simulink model "Demo"  (R2021a)
settings: Solver=FixedStepDiscrete  StartTime=0.0  StopTime=10  FixedStep=0.005  RelTol=1e-3  EnableMultiTasking=on
PreLoadFcn:
  | disp(pwd)
PostLoadFcn:
  | c2000demoscallback(1)
undefined symbols (not defined in the file or in its folder): CommandConstEnable, CommandData, FrameData, MailBoxRx, MailBoxTx, SCIAReceivedComplete, StatusConstClose, StatusConstClosed, StatusConstError, StatusConstHoming, StatusConstIdle, StatusConstPaused, StatusConstReady, StatusConstReset, StatusConstRunning, StatusConstStart, StatusConstStopped, StatusData
libraries: simulink x28, c280xlib x19, idelinklib_common x16, c2000lib x1, pid_lib x1, c2833xlib x1
(part 1 of 3)
settings Model: DataDictionary=DataD1.sldd  EnableAccessToBaseWorkspace=off  ExtModeTrigDuration=8  OrderedModelArguments=off  Creator=The MathWorks Inc.  LastModifiedBy=1
settings SolverCC: AlgebraicLoopSolver=TrustRegion
settings DataIOCC: LimitDataPoints=on  SaveFormat=Array  SignalLoggingSaveFormat=ModelDataLogs  SaveOutput=off  SaveTime=off  ReturnWorkspaceOutputs=off  SignalLoggingName=sigsOut
settings OptimizationCC: DefaultParameterBehavior=Inlined  DefaultUnderspecifiedDataType=single  PassReuseOutputArgsAs=Individual arguments  ExpressionDepthLimit=2147483647  InitFltsAndDblsToZero=on  LifeSpan=inf  MaxStackSize=512  EfficientTunableParamExpr=on
settings DebuggingCC: UnderspecifiedInitializationDetection=Classic  MergeDetectMultiDrivingBlocksExec=none  CheckExecutionContextPreStartOutputMsg=on  SignalResolutionControl=TryResolveAllWithWarning  MultiTaskDSMMsg=warning  MultiTaskCondExecSysMsg=none  SigSpecEnsureSampleTimeMsg=none  FcnCallInpInsideContextMsg=warning  StateNameClashWarn=warning  SFUnexpectedBacktrackingDiag=warning  SFNoUnconditionalDefaultTransitionDiag=warning  SFExecutionAtInitializationDiag=none  SFMachineParentedDataDiag=warning  ArithmeticOperatorsInVariantConditions=warning
settings HardwareCC: ProdBitPerChar=16  ProdBitPerInt=16  ProdBitPerPointer=32  ProdBitPerSizeT=32  ProdBitPerPtrDiffT=32  ProdLargestAtomicInteger=Integer  ProdLargestAtomicFloat=None  ProdWordSize=16  ProdLongLongMode=on  ProdHWDeviceType=Texas Instruments->C2000  TargetBitPerChar=16  TargetBitPerInt=16  TargetLargestAtomicInteger=Integer  TargetIntDivRoundTo=Zero  TargetEndianess=LittleEndian  TargetWordSize=16  TargetHWDeviceType=Texas Instruments->C2000  ProdEqTarget=off
settings ModelReferenceCC: UpdateModelReferenceTargets=IfOutOfDate  PropagateSignalLabelsOutOfModel=off
settings SFSimCC: SimUseLocalCustomCode=off  MATLABDynamicMemAlloc=off  CustomCodeUndefinedFunction=UseInterfaceOnly
settings RTWCC: SystemTargetFile=ert.tlc  HardwareBoard=TI Delfino F2833x  TemplateMakefile=ert_default_tmf  GenerateReport=on  RTWUseLocalCustomCode=off  Toolchain=Texas Instruments Code Composer Studio (C2000)  IncludeHyperlinkInReport=on  LaunchReport=on  GenerateTraceInfo=on  GenerateTraceReportSl=on  GenerateTraceReportSf=on  GenerateWebview=on
settings CodeAppCC: IgnoreCustomStorageClasses=off  SimulinkDataObjDesc=on  SFDataObjDesc=on  CustomSymbolStrType=$N$R$M  InsertBlockDesc=on  StateflowObjectComments=on  MATLABSourceComments=on  InternalIdentifier=Classic
settings ERTTargetCC: CodeReplacementLibrary=TI C28x  MultiwordLength=2048  ParMdlRefBuildCompliant=off  CPPClassGenCompliant=off  ConvertIfToSwitch=off  SuppressUnreachableDefaultCases=off
settings ConfigComp: CovMetricSettings=dw  CovSaveCumulativeToWorkspaceVar=on  CovSaveSingleToWorkspaceVar=on  CovExternalEMLEnable=off  CovSFcnEnable=off  PSAutoStubLUT=on

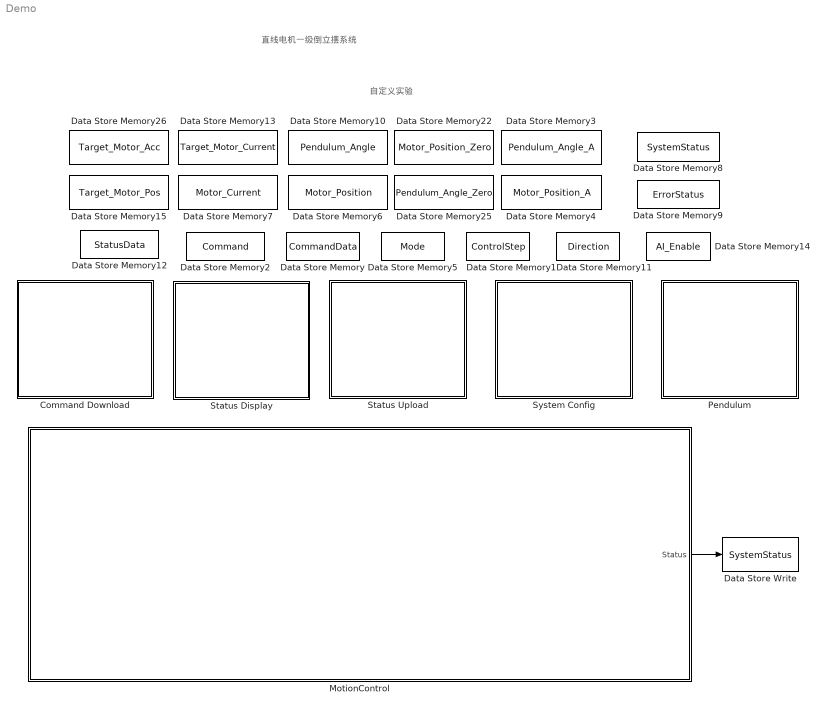
== system Demo ==
  note: 直线电机一级倒立摆系统
  note: 自定义实验
  Command Download : Subsystem  TreatAsAtomicUnit=on
  Data Store Memory11 : DataStoreMemory  DataStoreName=Direction  ReadBeforeWriteMsg=warning  WriteAfterWriteMsg=warning  WriteAfterReadMsg=warning  ShowAdditionalParam=off
  Data Store Memory14 : DataStoreMemory  DataStoreName=AI_Enable  ReadBeforeWriteMsg=warning  WriteAfterWriteMsg=warning  WriteAfterReadMsg=warning  InitialValue=1  ShowAdditionalParam=off  OutDataTypeStr=uint16
  Data Store Memory8 : DataStoreMemory  DataStoreName=SystemStatus  ReadBeforeWriteMsg=warning  WriteAfterWriteMsg=warning  WriteAfterReadMsg=warning  ShowAdditionalParam=off  OutDataTypeStr=uint16
  Data Store Memory9 : DataStoreMemory  DataStoreName=ErrorStatus  ReadBeforeWriteMsg=warning  WriteAfterWriteMsg=warning  WriteAfterReadMsg=warning  ShowAdditionalParam=off  OutDataTypeStr=uint16
  Data Store Write : DataStoreWrite  DataStoreName=SystemStatus  IndexOptions=Index vector (dialog)  Indices=1  OutputSizes=1
  Data Store Memory : DataStoreMemory  DataStoreName=CommandData  ReadBeforeWriteMsg=warning  WriteAfterWriteMsg=warning  WriteAfterReadMsg=warning  InitialValue=zeros(1,8)  ShowAdditionalParam=off  OutDataTypeStr=double
  Data Store Memory1 : DataStoreMemory  DataStoreName=ControlStep  ReadBeforeWriteMsg=warning  WriteAfterWriteMsg=warning  WriteAfterReadMsg=warning  ShowAdditionalParam=off  OutDataTypeStr=uint16
  Data Store Memory10 : DataStoreMemory  DataStoreName=Pendulum_Angle  ReadBeforeWriteMsg=warning  WriteAfterWriteMsg=warning  WriteAfterReadMsg=warning  ShowAdditionalParam=off  OutDataTypeStr=double
  Data Store Memory12 : DataStoreMemory  DataStoreName=StatusData  ReadBeforeWriteMsg=warning  WriteAfterWriteMsg=warning  WriteAfterReadMsg=warning  InitialValue=[0 0 0 0 0 0 0 0]  ShowAdditionalParam=off
  Data Store Memory13 : DataStoreMemory  DataStoreName=Target_Motor_Current  ReadBeforeWriteMsg=warning  WriteAfterWriteMsg=warning  WriteAfterReadMsg=warning  ShowAdditionalParam=off
  Data Store Memory15 : DataStoreMemory  DataStoreName=Target_Motor_Pos  ReadBeforeWriteMsg=warning  WriteAfterWriteMsg=warning  WriteAfterReadMsg=warning  ShowAdditionalParam=off
  Data Store Memory2 : DataStoreMemory  DataStoreName=Command  ReadBeforeWriteMsg=warning  WriteAfterWriteMsg=warning  WriteAfterReadMsg=warning  ShowAdditionalParam=off  OutDataTypeStr=uint16
  Data Store Memory22 : DataStoreMemory  DataStoreName=Motor_Position_Zero  ReadBeforeWriteMsg=warning  WriteAfterWriteMsg=warning  WriteAfterReadMsg=warning  ShowAdditionalParam=off  OutDataTypeStr=double
  Data Store Memory25 : DataStoreMemory  DataStoreName=Pendulum_Angle_Zero  ReadBeforeWriteMsg=warning  WriteAfterWriteMsg=warning  WriteAfterReadMsg=warning  ShowAdditionalParam=off  OutDataTypeStr=double
  Data Store Memory26 : DataStoreMemory  DataStoreName=Target_Motor_Acc  ReadBeforeWriteMsg=warning  WriteAfterWriteMsg=warning  WriteAfterReadMsg=warning  ShowAdditionalParam=off
  Data Store Memory3 : DataStoreMemory  DataStoreName=Pendulum_Angle_A  ReadBeforeWriteMsg=warning  WriteAfterWriteMsg=warning  WriteAfterReadMsg=warning  ShowAdditionalParam=off  OutDataTypeStr=double
  Data Store Memory4 : DataStoreMemory  DataStoreName=Motor_Position_A  ReadBeforeWriteMsg=warning  WriteAfterWriteMsg=warning  WriteAfterReadMsg=warning  ShowAdditionalParam=off  OutDataTypeStr=double
  Data Store Memory5 : DataStoreMemory  DataStoreName=Mode  ReadBeforeWriteMsg=warning  WriteAfterWriteMsg=warning  WriteAfterReadMsg=warning  ShowAdditionalParam=off  OutDataTypeStr=uint16
  Data Store Memory6 : DataStoreMemory  DataStoreName=Motor_Position  ReadBeforeWriteMsg=warning  WriteAfterWriteMsg=warning  WriteAfterReadMsg=warning  ShowAdditionalParam=off  OutDataTypeStr=double
  Data Store Memory7 : DataStoreMemory  DataStoreName=Motor_Current  ReadBeforeWriteMsg=warning  WriteAfterWriteMsg=warning  WriteAfterReadMsg=warning  ShowAdditionalParam=off
  MotionControl : Stateflow chart  TreatAsAtomicUnit=on
  Pendulum : Subsystem
  Status Display : Subsystem  TreatAsAtomicUnit=on
      settings: RTWSystemCode=Nonreusable function
  Status Upload : Subsystem  TreatAsAtomicUnit=on
  System Config : Subsystem  TreatAsAtomicUnit=on
  wires:
  MotionControl/1(Status) -> Data Store Write/1

== system Demo/Command Download ==
  Data Store Memory12 : DataStoreMemory  DataStoreName=FrameData  ReadBeforeWriteMsg=warning  WriteAfterWriteMsg=warning  WriteAfterReadMsg=warning  InitialValue=zeros(1,17)  ShowAdditionalParam=off  OutDataTypeStr=uint16
  SCIA_Interrupt : c2000lib/Scheduling/C28x Hardware Interrupt  irqnumbers=9  pienumbers=1  irqpriorities=0  irqpreempts=0  showinput=off  dspchiptype=C280X
      settings: SourceProductBaseCode=TIC2000
  SCIA_RX_Process : Subsystem  TreatAsAtomicUnit=on
  wires:
  SCIA_Interrupt/1 -> SCIA_RX_Process/Trigger

== system Demo/MotionControl/Close ==
  f : TriggerPort  TriggerType=function-call  VariantControl=(inherit)
      settings: CopyFcn=Stateflow.SLINSF.SimulinkMan.removeBlockPreDeleteFcn  PreDeleteFcn=Stateflow.SLINSF.SimulinkMan.unsafePredeleteFcn
  Constant : Constant  OutDataTypeStr=uint16
  Constant1 : Constant  Value=0
  Constant2 : Constant  Value=0  OutDataTypeStr=uint16
  Constant5 : Constant  Value=StatusConstIdle
  Data Store Write : DataStoreWrite  DataStoreName=AI_Enable  IndexOptions=Index vector (dialog)  Indices=1  OutputSizes=1
  Data Store Write1 : DataStoreWrite  DataStoreName=Target_Motor_Current  IndexOptions=Index vector (dialog)  Indices=1  OutputSizes=1
  Data Store Write2 : DataStoreWrite  DataStoreName=Target_Motor_Acc  IndexOptions=Index vector (dialog)  Indices=1  OutputSizes=1
  Data Store Write3 : DataStoreWrite  DataStoreName=Mode  IndexOptions=Index vector (dialog)  Indices=1  OutputSizes=1
  MO : Constant  Value=[hex2dec('4F4D') 0 0 0]  OutDataTypeStr=uint16
  eCANA Transmit : Subsystem  TreatAsAtomicUnit=on  mask(eCANA Transimit Blocks){MailBoxTx=1, MailBoxRx=4}
      mask help: eCANA MailBox Transimit
      mask DialogControl ParameterGroup Prompt: Parameter Setting
  Status : Outport  OutDataTypeStr=uint16  PortDimensions=[1 1]  VectorParamsAs1DForOutWhenUnconnected=off
  wires:
  Constant1/1 -> Data Store Write2/1, Data Store Write1/1
  Constant5/1 -> Status/1
  Constant/1 -> Data Store Write/1
  MO/1 -> eCANA Transmit/1(DataTx)
  Constant2/1 -> Data Store Write3/1

== system Demo/MotionControl/Home ==
  f : TriggerPort  TriggerType=function-call  VariantControl=(inherit)
      settings: CopyFcn=Stateflow.SLINSF.SimulinkMan.removeBlockPreDeleteFcn  PreDeleteFcn=Stateflow.SLINSF.SimulinkMan.unsafePredeleteFcn
  Add : Sum
  Compare To Constant1 : simulink/Logic and Bit Operations/Compare To Constant  relop=>=  const=uint16(15)  OutDataTypeStr=boolean
  Constant : Constant  Value=StatusConstHoming
  Constant1 : Constant  Value=StatusConstReady
  Data Store Read2 : DataStoreRead  DataStoreName=ControlStep  IndexOptions=Index vector (dialog)  Indices=1  OutputSizes=1
  PX : Subsystem  TreatAsAtomicUnit=on
  ResetAngle : Subsystem  TreatAsAtomicUnit=on
  Switch : Switch  Criteria=u2 > Threshold  Threshold=uint16(0)
  Switch Case : SwitchCase  CaseConditions={1,2,3,4}
  TForAI0 : Subsystem  TreatAsAtomicUnit=on
  TForAI1 : Subsystem  TreatAsAtomicUnit=on
  Status : Outport  OutDataTypeStr=uint16  PortDimensions=1
  wires:
  Switch Case/2 -> TForAI1/Action
  Constant/1 -> Add/1
  Switch Case/1 -> ResetAngle/Action
  Compare To Constant1/1 -> Switch/2
  Data Store Read2/1 -> Switch Case/1, Add/2, Compare To Constant1/1
  Add/1 -> Switch/3
  Constant1/1 -> Switch/1
  Switch Case/3 -> PX/Action
  Switch/1 -> Status/1
  Switch Case/4 -> TForAI0/Action

== system Demo/MotionControl/Idle ==
  f : TriggerPort  TriggerType=function-call  VariantControl=(inherit)
      settings: CopyFcn=Stateflow.SLINSF.SimulinkMan.removeBlockPreDeleteFcn  PreDeleteFcn=Stateflow.SLINSF.SimulinkMan.unsafePredeleteFcn
  Constant4 : Constant  Value=StatusConstReset
  Constant5 : Constant  Value=StatusConstStart
  Constant6 : Constant  Value=StatusConstIdle
  Data Store Read : DataStoreRead  DataStoreName=Command  IndexOptions=Index vector (dialog)  Indices=1  OutputSizes=1
  Index Vector : MultiPortSwitch  DataPortOrder=Specify indices  Inputs=1  DataPortIndices={CommandConstStart,CommandConstReset}  DataPortForDefault=Additional data port  DiagnosticForDefault=None
  Status : Outport  OutDataTypeStr=uint16  PortDimensions=[1 1]
  wires:
  Index Vector/1 -> Status/1
  Constant4/1 -> Index Vector/3
  Constant5/1 -> Index Vector/2
  Data Store Read/1 -> Index Vector/1
  Constant6/1 -> Index Vector/4

== system Demo/MotionControl/Initial ==
  f : TriggerPort  TriggerType=function-call  VariantControl=(inherit)
      settings: CopyFcn=Stateflow.SLINSF.SimulinkMan.removeBlockPreDeleteFcn  PreDeleteFcn=Stateflow.SLINSF.SimulinkMan.unsafePredeleteFcn
  Bus Assignment : BusAssignment  Priority=1  AssignedSignals=MailBoxTx,MailBoxRx
  Bus Assignment1 : BusAssignment  Priority=1  Commented=on  AssignedSignals=MailBoxTx,MailBoxRx
  Constant1 : Constant  Value=4  OutDataTypeStr=uint16  SampleTime=-1
  Constant2 : Constant  OutDataTypeStr=uint16  SampleTime=-1
  Constant3 : Constant  Commented=on  Value=5  OutDataTypeStr=uint16  SampleTime=-1
  Constant4 : Constant  Commented=on  Value=2  OutDataTypeStr=uint16  SampleTime=-1
  Data Store Read : DataStoreRead  DataStoreName=CanMsgA  IndexOptions=Index vector (dialog)  Indices=1  OutputSizes=1
  Data Store Read1 : DataStoreRead  Commented=on  DataStoreName=CanMsgA1  IndexOptions=Index vector (dialog)  Indices=1  OutputSizes=1
  Data Store Write : DataStoreWrite  DataStoreName=CanMsgA  IndexOptions=Index vector (dialog)  Indices=1  OutputSizes=1
  Data Store Write1 : DataStoreWrite  Commented=on  DataStoreName=CanMsgA1  IndexOptions=Index vector (dialog)  Indices=1  OutputSizes=1
  wires:
  Constant2/1 -> Bus Assignment/2
  Constant1/1 -> Bus Assignment/3
  Bus Assignment/1 -> Data Store Write/1
  Data Store Read/1 -> Bus Assignment/1
  Data Store Read1/1 -> Bus Assignment1/1
  Bus Assignment1/1 -> Data Store Write1/1
  Constant3/1 -> Bus Assignment1/3
  Constant4/1 -> Bus Assignment1/2

== system Demo/MotionControl/Ready ==
  f : TriggerPort  TriggerType=function-call  VariantControl=(inherit)
      settings: CopyFcn=Stateflow.SLINSF.SimulinkMan.removeBlockPreDeleteFcn  PreDeleteFcn=Stateflow.SLINSF.SimulinkMan.unsafePredeleteFcn
  Constant1 : Constant  Value=StatusConstHoming
  Constant2 : Constant  Value=StatusConstRunning
  Constant3 : Constant  Value=StatusConstReady
  Constant4 : Constant  Value=StatusConstClose
  Data Store Read : DataStoreRead  DataStoreName=Command  IndexOptions=Index vector (dialog)  Indices=1  OutputSizes=1
  Multiport Switch : MultiPortSwitch  DataPortOrder=Specify indices  DataPortIndices={CommandConstHome,CommandConstRun,CommandConstDisable}  DataPortForDefault=Additional data port  DiagnosticForDefault=None
  Status : Outport  OutDataTypeStr=uint16  PortDimensions=1
  wires:
  Data Store Read/1 -> Multiport Switch/1
  Constant2/1 -> Multiport Switch/3
  Constant1/1 -> Multiport Switch/2
  Multiport Switch/1 -> Status/1
  Constant3/1 -> Multiport Switch/5
  Constant4/1 -> Multiport Switch/4

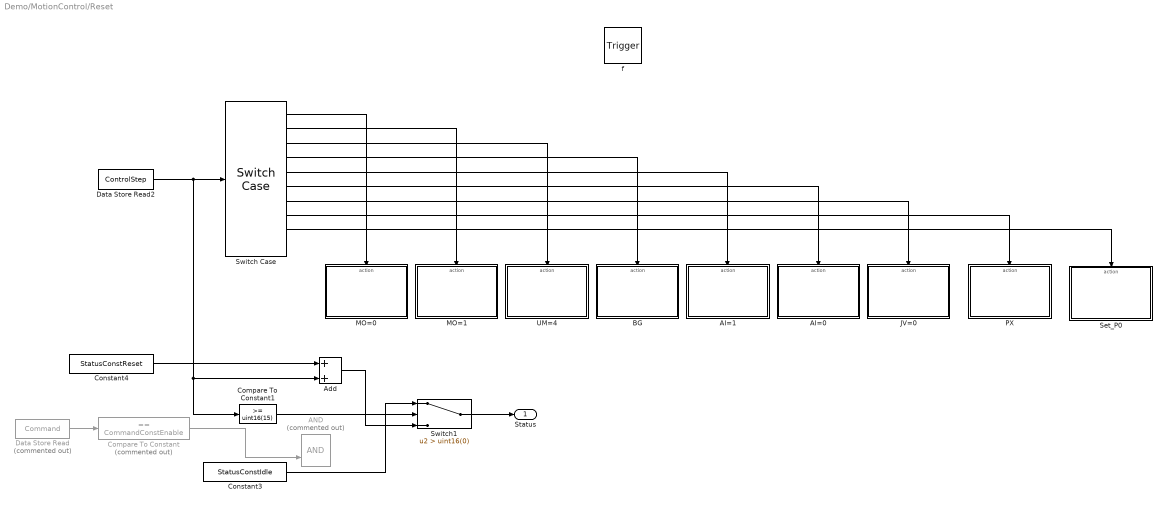
== system Demo/MotionControl/Reset ==
  f : TriggerPort  TriggerType=function-call  VariantControl=(inherit)
      settings: CopyFcn=Stateflow.SLINSF.SimulinkMan.removeBlockPreDeleteFcn  PreDeleteFcn=Stateflow.SLINSF.SimulinkMan.unsafePredeleteFcn
  AI=0 : Subsystem  TreatAsAtomicUnit=on
  AI=1 : Subsystem  TreatAsAtomicUnit=on
  AND : Logic  Commented=on  AllPortsSameDT=off  OutDataTypeStr=boolean
  Add : Sum
  "BG " : Subsystem  TreatAsAtomicUnit=on
  Compare To Constant : simulink/Logic and Bit Operations/Compare To Constant  Commented=on  relop===  const=CommandConstEnable  OutDataTypeStr=boolean
  Compare To Constant1 : simulink/Logic and Bit Operations/Compare To Constant  relop=>=  const=uint16(15)  OutDataTypeStr=boolean
  Constant3 : Constant  Value=StatusConstIdle
  Constant4 : Constant  Value=StatusConstReset
  Data Store Read : DataStoreRead  Commented=on  DataStoreName=Command  IndexOptions=Index vector (dialog)  Indices=1  OutputSizes=1
  Data Store Read2 : DataStoreRead  DataStoreName=ControlStep  IndexOptions=Index vector (dialog)  Indices=1  OutputSizes=1
  JV=0 : Subsystem  TreatAsAtomicUnit=on
  MO=0 : Subsystem  TreatAsAtomicUnit=on
  MO=1 : Subsystem  TreatAsAtomicUnit=on
  PX : Subsystem  TreatAsAtomicUnit=on
  Set_P0 : Subsystem  TreatAsAtomicUnit=on
  Switch Case : SwitchCase  CaseConditions={1,2,3,4,5,6,7,8,9}
  Switch1 : Switch  Criteria=u2 > Threshold  Threshold=uint16(0)
  UM=4 : Subsystem  TreatAsAtomicUnit=on
  Status : Outport  OutDataTypeStr=uint16  PortDimensions=1
  wires:
  Data Store Read2/1 -> Compare To Constant1/1, Add/2, Switch Case/1
  Switch Case/1 -> MO=0/Action
  Switch Case/2 -> MO=1/Action
  Switch Case/3 -> UM=4/Action
  Switch Case/5 -> AI=1/Action
  Switch Case/6 -> AI=0/Action
  Switch Case/4 -> "BG "/Action
  Switch Case/7 -> JV=0/Action
  Constant4/1 -> Add/1
  Switch1/1 -> Status/1
  Add/1 -> Switch1/3
  Constant3/1 -> Switch1/1
  Data Store Read/1 -> Compare To Constant/1
  Compare To Constant/1 -> AND/2
  Compare To Constant1/1 -> Switch1/2
  Switch Case/8 -> PX/Action
  Switch Case/9 -> Set_P0/Action

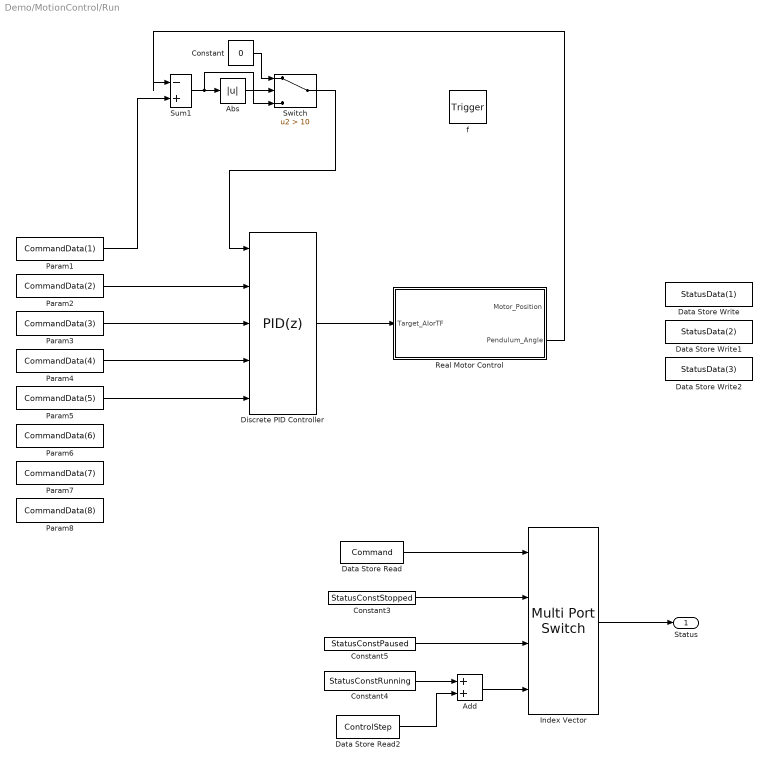
== system Demo/MotionControl/Run ==
  f : TriggerPort  TriggerType=function-call  VariantControl=(inherit)
      settings: CopyFcn=Stateflow.SLINSF.SimulinkMan.removeBlockPreDeleteFcn  PreDeleteFcn=Stateflow.SLINSF.SimulinkMan.unsafePredeleteFcn
  Abs : Abs
  Add : Sum
  Constant : Constant  Value=0
  Constant3 : Constant  Value=StatusConstStopped
  Constant4 : Constant  Value=StatusConstRunning
  Constant5 : Constant  Value=StatusConstPaused
  Data Store Read : DataStoreRead  DataStoreName=Command  IndexOptions=Index vector (dialog)  Indices=1  OutputSizes=1
  Data Store Read2 : DataStoreRead  DataStoreName=ControlStep  IndexOptions=Index vector (dialog)  Indices=1  OutputSizes=1
  Data Store Write : DataStoreWrite  DataStoreName=StatusData  DataStoreElements=StatusData(1)  IndexOptions=Index vector (dialog)  Indices=1  OutputSizes=1
  Data Store Write1 : DataStoreWrite  DataStoreName=StatusData  DataStoreElements=StatusData(2)  IndexOptions=Index vector (dialog)  Indices=1  OutputSizes=1
  Data Store Write2 : DataStoreWrite  DataStoreName=StatusData  DataStoreElements=StatusData(3)  IndexOptions=Index vector (dialog)  Indices=1  OutputSizes=1
  Discrete PID Controller : pid_lib/PID Controller  Controller=PID  Form=Parallel  TimeDomain=Discrete-time  UseExternalTs=off  SampleTime=-1  IntegratorMethod=Forward Euler  FilterMethod=Forward Euler  ControllerParametersSource=external  P=1  I=1  D=0  UseFilter=on  N=100  TunerSelectOption=Transfer Function Based (PID Tuner App)  InitialConditionSource=internal  InitialConditionForIntegrator=0  InitialConditionForFilter=0  DifferentiatorICPrevScaledInput=0  ExternalReset=none  TrackingMode=off  Kt=1  LimitOutput=off  SatLimitsSource=internal  UpperSaturationLimit=inf  LowerSaturationLimit=-inf  LinearizeAsGain=off  AntiWindupMode=none  Kb=1  POutMin=[]  POutMax=[]  IOutMin=[]  IOutMax=[]  DOutMin=[]  DOutMax=[]  NOutMin=[]  NOutMax=[]  SumOutMin=[]  SumOutMax=[]  SaturationOutMin=[]  SaturationOutMax=[]  PParamMin=[]  PParamMax=[]  IParamMin=[]  IParamMax=[]  DParamMin=[]  DParamMax=[]  NParamMin=[]  NParamMax=[]  KbParamMin=[]  KbParamMax=[]  KtParamMin=[]  KtParamMax=[]  KbOutMin=[]  KbOutMax=[]  KtOutMin=[]  KtOutMax=[]  IntegratorOutMin=[]  IntegratorOutMax=[]  FilterOutMin=[]  FilterOutMax=[]  SumI1OutMin=[]  SumI1OutMax=[]  SumI2OutMin=[]  SumI2OutMax=[]  SumI3OutMin=[]  SumI3OutMax=[]  SumI4OutMin=[]  SumI4OutMax=[]  SumDOutMin=[]  SumDOutMax=[]  DifferentiatorOutMin=[]  DifferentiatorOutMax=[]  FilterDiffOutCoefMin=[]  FilterDiffOutCoefMax=[]  ReciprocalOutMin=[]  ReciprocalOutMax=[]  SumDenOutMin=[]  SumDenOutMax=[]  SumNumOutMin=[]  SumNumOutMax=[]  DivideOutMin=[]  DivideOutMax=[]  UdiffTsProdOutMin=[]  UdiffTsProdOutMax=[]  NTsProdOutMin=[]  NTsProdOutMax=[]  UintegralTsProdOutMin=[]  UintegralTsProdOutMax=[]  UngainTsProdOutMin=[]  UngainTsProdOutMax=[]  IntegratorContinuousStateAttributes=''  IntegratorStateMustResolveToSignalObject=off  IntegratorRTWStateStorageClass=Auto  FilterContinuousStateAttributes=''  FilterStateMustResolveToSignalObject=off  FilterRTWStateStorageClass=Auto  ParallelPVariant=ExternalParameters  IdealPVariant=Disabled  IVariant=ExternalParameters  DVariant=ExternalParameters  IntegratorVariant=Discrete  SatVariant=Disabled  AWVariant=Passthrough  PCopyVariant=Disabled  TRVariant=Disabled  FdbkBlocksVariant=Forward  IdealPFdbkVariant=Disabled  SatFdbkVariant=Disabled  DerivativeFilterVariant=ForwardEulerFilter  NVariant=ExternalParameters  NCopyVariant=Disabled  FilterICVariant=InternalICsFilter  IntegratorICVariant=InternalICs  ExternalResetVariant=Disabled  TRSumVariant=Passthrough  SumFdbkVariant=Disabled  SumVariant=Sum_PID  TsampFilterVariant=InternalTs  TsampNgainVariant=Passthrough  TsampIntegralVariant=Passthrough  ExternalSaturationOutDataTypeStr=Inherit: Same as second input
  Index Vector : MultiPortSwitch  DataPortOrder=Specify indices  Inputs=1  DataPortIndices={CommandConstStop,CommandConstPause}  DataPortForDefault=Additional data port  DiagnosticForDefault=None
  Param1 : DataStoreRead  DataStoreName=CommandData  DataStoreElements=CommandData(1)  IndexOptions=Index vector (dialog)  Indices=1  OutputSizes=1
  Param2 : DataStoreRead  DataStoreName=CommandData  DataStoreElements=CommandData(2)  IndexOptions=Index vector (dialog)  Indices=1  OutputSizes=1
  Param3 : DataStoreRead  DataStoreName=CommandData  DataStoreElements=CommandData(3)  IndexOptions=Index vector (dialog)  Indices=1  OutputSizes=1
  Param4 : DataStoreRead  DataStoreName=CommandData  DataStoreElements=CommandData(4)  IndexOptions=Index vector (dialog)  Indices=1  OutputSizes=1
  Param5 : DataStoreRead  DataStoreName=CommandData  DataStoreElements=CommandData(5)  IndexOptions=Index vector (dialog)  Indices=1  OutputSizes=1
  Param6 : DataStoreRead  DataStoreName=CommandData  DataStoreElements=CommandData(6)  IndexOptions=Index vector (dialog)  Indices=1  OutputSizes=1
  Param7 : DataStoreRead  DataStoreName=CommandData  DataStoreElements=CommandData(7)  IndexOptions=Index vector (dialog)  Indices=1  OutputSizes=1
  Param8 : DataStoreRead  DataStoreName=CommandData  DataStoreElements=CommandData(8)  IndexOptions=Index vector (dialog)  Indices=1  OutputSizes=1
  Real Motor Control : Subsystem
  Sum1 : Sum  Inputs=|-+
  Switch : Switch  Criteria=u2 > Threshold  Threshold=10
  Status : Outport  OutDataTypeStr=uint16  PortDimensions=[1 1]  VectorParamsAs1DForOutWhenUnconnected=off
  wires:
  Constant5/1 -> Index Vector/3
  Data Store Read/1 -> Index Vector/1
  Constant3/1 -> Index Vector/2
  Constant4/1 -> Add/1
  Index Vector/1 -> Status/1
  Add/1 -> Index Vector/4
  Data Store Read2/1 -> Add/2
  Discrete PID Controller/1 -> Real Motor Control/1(Target_AIorTF)
  Sum1/1 -> Switch/3, Abs/1
  Real Motor Control/2(Pendulum_Angle) -> Sum1/1
  Abs/1 -> Switch/2
  Constant/1 -> Switch/1
  Switch/1 -> Discrete PID Controller/1
  Param1/1 -> Sum1/2
  Param2/1 -> Discrete PID Controller/2
  Param3/1 -> Discrete PID Controller/3
  Param4/1 -> Discrete PID Controller/4
  Param5/1 -> Discrete PID Controller/5

== system Demo/MotionControl/Start ==
  f : TriggerPort  TriggerType=function-call  VariantControl=(inherit)
      settings: CopyFcn=Stateflow.SLINSF.SimulinkMan.removeBlockPreDeleteFcn  PreDeleteFcn=Stateflow.SLINSF.SimulinkMan.unsafePredeleteFcn
  Add : Sum
  BG : Subsystem  TreatAsAtomicUnit=on
  Compare To Constant1 : simulink/Logic and Bit Operations/Compare To Constant  relop=>=  const=uint16(15)  OutDataTypeStr=boolean
  Constant : Constant  Value=StatusConstStart
  Constant1 : Constant  Value=StatusConstReady
  Data Store Read2 : DataStoreRead  DataStoreName=ControlStep  IndexOptions=Index vector (dialog)  Indices=1  OutputSizes=1
  MO=1 : Subsystem  TreatAsAtomicUnit=on
  Switch : Switch  Criteria=u2 > Threshold  Threshold=uint16(0)
  Switch Case : SwitchCase  CaseConditions={1,2,3}
  UM=1or4 : Subsystem  TreatAsAtomicUnit=on
  Status : Outport  OutDataTypeStr=uint16  PortDimensions=1
  wires:
  Switch Case/2 -> UM=1or4/Action
  Switch Case/3 -> BG/Action
  Compare To Constant1/1 -> Switch/2
  Add/1 -> Switch/3
  Constant1/1 -> Switch/1
  Switch/1 -> Status/1
  Data Store Read2/1 -> Switch Case/1, Add/1, Compare To Constant1/1
  Switch Case/1 -> MO=1/Action
  Constant/1 -> Add/2

== system Demo/MotionControl/Stop ==
  f : TriggerPort  TriggerType=function-call  VariantControl=(inherit)
      settings: CopyFcn=Stateflow.SLINSF.SimulinkMan.removeBlockPreDeleteFcn  PreDeleteFcn=Stateflow.SLINSF.SimulinkMan.unsafePredeleteFcn
  Constant : Constant  OutDataTypeStr=uint16
  Constant1 : Constant  Value=0
  Constant5 : Constant  Value=StatusConstReady
  Data Store Write : DataStoreWrite  DataStoreName=AI_Enable  IndexOptions=Index vector (dialog)  Indices=1  OutputSizes=1
  Data Store Write1 : DataStoreWrite  DataStoreName=Target_Motor_Current  IndexOptions=Index vector (dialog)  Indices=1  OutputSizes=1
  Data Store Write2 : DataStoreWrite  DataStoreName=Target_Motor_Acc  IndexOptions=Index vector (dialog)  Indices=1  OutputSizes=1
  Status : Outport  OutDataTypeStr=uint16  PortDimensions=[1 1]  VectorParamsAs1DForOutWhenUnconnected=off
  wires:
  Constant5/1 -> Status/1
  Constant/1 -> Data Store Write/1
  Constant1/1 -> Data Store Write2/1, Data Store Write1/1

== system Demo/Pendulum ==
  note: 采集滑块位置信息
  note: 采集摆杆角度信息
  Subsystem : Subsystem  Priority=1  TreatAsAtomicUnit=on
  Subsystem1 : Subsystem

== system Demo/Status Display ==
  note: 如果状态发生切换，才进行显示
  CTC : simulink/Logic and Bit Operations/Compare To Constant  relop=<=  const=200  OutDataTypeStr=boolean
  Counter : simulink/Sources/Counter Limited  uplimit=400  tsamp=-1
  Data Store Read1 : DataStoreRead  DataStoreName=SystemStatus  IndexOptions=Index vector (dialog)  Indices=1  OutputSizes=1
  Data Store Read8 : DataStoreRead  DataStoreName=ErrorStatus  IndexOptions=Index vector (dialog)  Indices=1  OutputSizes=1
  Delay : Delay  DelayLength=1
  Enabled Subsystem : Subsystem  TreatAsAtomicUnit=on
  GPIO28 : c2833xlib/Digital Output  GPIO_Number=GPIO24~GPIO31  GPIO_Bit0=off  GPIO_BIT0_Toggle=off  GPIO_Bit1=off  GPIO_BIT1_Toggle=off  GPIO_Bit2=off  GPIO_BIT2_Toggle=off  GPIO_Bit3=off  GPIO_BIT3_Toggle=off  GPIO_Bit4=on  GPIO_BIT4_Toggle=off  GPIO_Bit5=off  GPIO_BIT5_Toggle=off  GPIO_Bit6=off  GPIO_BIT6_Toggle=off  GPIO_Bit7=off  GPIO_BIT7_Toggle=off
      settings: SourceProductBaseCode=TIC2000
  Relational Operator1 : RelationalOperator  Operator=~=  OutDataTypeStr=boolean  RndMeth=Simplest
  wires:
  Counter/1 -> CTC/1
  CTC/1 -> GPIO28/1
  Relational Operator1/1 -> Enabled Subsystem/Enable
  Data Store Read8/1 -> Enabled Subsystem/2(Status2)
  Data Store Read1/1 -> Relational Operator1/2, Enabled Subsystem/1(Status1), Delay/1
  Delay/1 -> Relational Operator1/1

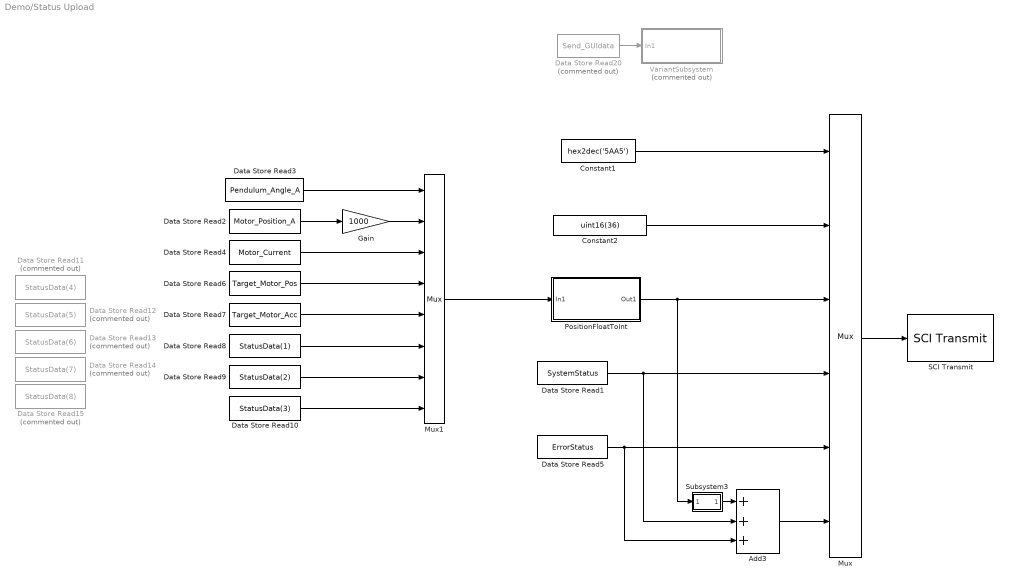
== system Demo/Status Upload ==
  Add3 : Sum  Inputs=+++
  Constant1 : Constant  Value=hex2dec('5AA5')  OutDataTypeStr=uint16  SampleTime=-1
  Constant2 : Constant  Value=uint16(36)
  Data Store Read1 : DataStoreRead  DataStoreName=SystemStatus  IndexOptions=Index vector (dialog)  Indices=1  OutputSizes=1
  Data Store Read10 : DataStoreRead  DataStoreName=StatusData  DataStoreElements=StatusData(3)  IndexOptions=Index vector (dialog)  Indices=1  OutputSizes=1
  Data Store Read11 : DataStoreRead  Commented=on  DataStoreName=StatusData  DataStoreElements=StatusData(4)  IndexOptions=Index vector (dialog)  Indices=1  OutputSizes=1
  Data Store Read12 : DataStoreRead  Commented=on  DataStoreName=StatusData  DataStoreElements=StatusData(5)  IndexOptions=Index vector (dialog)  Indices=1  OutputSizes=1
  Data Store Read13 : DataStoreRead  Commented=on  DataStoreName=StatusData  DataStoreElements=StatusData(6)  IndexOptions=Index vector (dialog)  Indices=1  OutputSizes=1
  Data Store Read14 : DataStoreRead  Commented=on  DataStoreName=StatusData  DataStoreElements=StatusData(7)  IndexOptions=Index vector (dialog)  Indices=1  OutputSizes=1
  Data Store Read15 : DataStoreRead  Commented=on  DataStoreName=StatusData  DataStoreElements=StatusData(8)  IndexOptions=Index vector (dialog)  Indices=1  OutputSizes=1
  Data Store Read2 : DataStoreRead  DataStoreName=Motor_Position_A  IndexOptions=Index vector (dialog)  Indices=1  OutputSizes=1
  Data Store Read20 : DataStoreRead  Commented=on  DataStoreName=Send_GUIdata  IndexOptions=Index vector (dialog)  Indices=1  OutputSizes=1
  Data Store Read3 : DataStoreRead  DataStoreName=Pendulum_Angle_A  IndexOptions=Index vector (dialog)  Indices=1  OutputSizes=1
  Data Store Read4 : DataStoreRead  DataStoreName=Motor_Current  IndexOptions=Index vector (dialog)  Indices=1  OutputSizes=1
  Data Store Read5 : DataStoreRead  DataStoreName=ErrorStatus  IndexOptions=Index vector (dialog)  Indices=1  OutputSizes=1
  Data Store Read6 : DataStoreRead  DataStoreName=Target_Motor_Pos  IndexOptions=Index vector (dialog)  Indices=1  OutputSizes=1
  Data Store Read7 : DataStoreRead  DataStoreName=Target_Motor_Acc  IndexOptions=Index vector (dialog)  Indices=1  OutputSizes=1
  Data Store Read8 : DataStoreRead  DataStoreName=StatusData  DataStoreElements=StatusData(1)  IndexOptions=Index vector (dialog)  Indices=1  OutputSizes=1
  Data Store Read9 : DataStoreRead  DataStoreName=StatusData  DataStoreElements=StatusData(2)  IndexOptions=Index vector (dialog)  Indices=1  OutputSizes=1
  Gain : Gain  Gain=1000
  Mux : Mux  Inputs=6
  Mux1 : Mux  Inputs=8
  PositionFloatToInt : Subsystem
  SCI Transmit : c280xlib/SCI Transmit  sciModule=A  dataHead=''  dataTail=''  postInterrupt=off  numFifo=10
  Subsystem3 : Subsystem
  VariantSubsystem : Subsystem  Commented=on  Variant=on  VariantControlMode=label  LabelModeActiveChoice=Variant1
  wires:
  Data Store Read20/1 -> VariantSubsystem/1(In1)
  Add3/1 -> Mux/6
  Data Store Read1/1 -> Add3/2, Mux/4
  Subsystem3/1(Out1) -> Add3/1
  Constant1/1 -> Mux/1
  Data Store Read5/1 -> Add3/3, Mux/5
  Constant2/1 -> Mux/2
  Mux1/1 -> PositionFloatToInt/1(In1)
  PositionFloatToInt/1(Out1) -> Subsystem3/1(In1), Mux/3
  Mux/1 -> SCI Transmit/1
  Data Store Read6/1 -> Mux1/4
  Gain/1 -> Mux1/2
  Data Store Read3/1 -> Mux1/1
  Data Store Read4/1 -> Mux1/3
  Data Store Read2/1 -> Gain/1
  Data Store Read7/1 -> Mux1/5
  Data Store Read10/1 -> Mux1/8
  Data Store Read9/1 -> Mux1/7
  Data Store Read8/1 -> Mux1/6

== system Demo/System Config ==
  CAN_Config_C : Subsystem  Commented=on
  CAN_Config_S : Subsystem
  HC595_Config : Subsystem  Commented=on
  LCD_Config : Subsystem
  SCI_Config : Subsystem

== system Demo/Command Download/SCIA_RX_Process ==
  SCIA_RX_ISA : TriggerPort  TriggerType=function-call  VariantControl=Variant
  Process : Subsystem  Priority=2  TreatAsAtomicUnit=on
  Receive : Subsystem  Priority=1  TreatAsAtomicUnit=on

== system Demo/MotionControl/Close/eCANA Transmit ==
  DataTx : Inport
  Bus Assignment : BusAssignment  Priority=1  AssignedSignals=TxWord
  Data Store Read : DataStoreRead  DataStoreName=CanMsgA  IndexOptions=Index vector (dialog)  Indices=1  OutputSizes=1
  Data Store Write : DataStoreWrite  DataStoreName=CanMsgA  IndexOptions=Index vector (dialog)  Indices=1  OutputSizes=1
  System Outputs : Subsystem  Priority=2  mask(System Outputs){MailBox=0}
      settings: CopyFcn=cccopyfcn(gcb)  OpenFcn=ccopenfcn('System Outputs Function')
      mask Help: eval('feval(''rtwprivate'',''rtwhelpview'',''rtw_sys_outputs_block'')');
      mask TypeOptions MailBox: 0 | 1 | 2 | 3 | 4 | 5
  wires:
  DataTx/1 -> Bus Assignment/2
  Data Store Read/1 -> Bus Assignment/1
  Bus Assignment/1 -> Data Store Write/1

== system Demo/MotionControl/Home/PX ==
  Action Port : ActionPort  ActionPortLabel=case [ 3 ]:
  Add Constant : Bias  Bias=uint16(1)
  Add1 : Sum  Inputs=+-
  Add3 : Sum  Inputs=-+
  Data Store Read : DataStoreRead  DataStoreName=ControlStep  IndexOptions=Index vector (dialog)  Indices=1  OutputSizes=1
  Data Store Read1 : DataStoreRead  DataStoreName=Motor_Position  IndexOptions=Index vector (dialog)  Indices=1  OutputSizes=1
  Data Store Read2 : DataStoreRead  DataStoreName=ControlStep  IndexOptions=Index vector (dialog)  Indices=1  OutputSizes=1
  Data Store Read3 : DataStoreRead  DataStoreName=Motor_Position_A  IndexOptions=Index vector (dialog)  Indices=1  OutputSizes=1
  Data Store Read4 : DataStoreRead  DataStoreName=Motor_Position_Zero  IndexOptions=Index vector (dialog)  Indices=1  OutputSizes=1
  Data Store Read5 : DataStoreRead  DataStoreName=Motor_Position_Zero  IndexOptions=Index vector (dialog)  Indices=1  OutputSizes=1
  Data Store Read6 : DataStoreRead  DataStoreName=Motor_Position  IndexOptions=Index vector (dialog)  Indices=1  OutputSizes=1
  Data Store Write : DataStoreWrite  DataStoreName=ControlStep  IndexOptions=Index vector (dialog)  Indices=1  OutputSizes=1
  Switch : Switch
  Switch1 : Switch  Criteria=u2 > Threshold
  wires:
  Data Store Read1/1 -> Add1/1
  Add Constant/1 -> Switch/1
  Add3/1 -> Switch1/3
  Switch1/1 -> Switch/2
  Data Store Read3/1 -> Switch1/2
  Data Store Read6/1 -> Add3/1
  Data Store Read5/1 -> Add3/2
  Data Store Read4/1 -> Add1/2
  Add1/1 -> Switch1/1
  Switch/1 -> Data Store Write/1
  Data Store Read/1 -> Switch/3
  Data Store Read2/1 -> Add Constant/1

== system Demo/MotionControl/Home/ResetAngle ==
  Action Port : ActionPort  ActionPortLabel=case [ 1 ]:
  Add Constant : Bias  Bias=uint16(1)
  Add Constant1 : Bias  Bias=180
  Constant : Constant  Value=-1
  Constant1 : Constant
  Constant2 : Constant  Value=uint16(0)
  Data Store Read : DataStoreRead  DataStoreName=Motor_Position_A  IndexOptions=Index vector (dialog)  Indices=1  OutputSizes=1
  Data Store Read1 : DataStoreRead  DataStoreName=Pendulum_Angle  IndexOptions=Index vector (dialog)  Indices=1  OutputSizes=1
  Data Store Read2 : DataStoreRead  DataStoreName=ControlStep  IndexOptions=Index vector (dialog)  Indices=1  OutputSizes=1
  Data Store Write : DataStoreWrite  DataStoreName=Command  IndexOptions=Index vector (dialog)  Indices=1  OutputSizes=1
  Data Store Write1 : DataStoreWrite  DataStoreName=Pendulum_Angle_Zero  IndexOptions=Index vector (dialog)  Indices=1  OutputSizes=1
  Data Store Write2 : DataStoreWrite  DataStoreName=ControlStep  IndexOptions=Index vector (dialog)  Indices=1  OutputSizes=1
  Data Store Write3 : DataStoreWrite  DataStoreName=Direction  IndexOptions=Index vector (dialog)  Indices=1  OutputSizes=1
  Switch : Switch  Criteria=u2 > Threshold
  wires:
  Data Store Read1/1 -> Add Constant1/1
  Add Constant/1 -> Data Store Write2/1
  Data Store Read2/1 -> Add Constant/1
  Add Constant1/1 -> Data Store Write1/1
  Constant2/1 -> Data Store Write/1
  Constant1/1 -> Switch/3
  Constant/1 -> Switch/1
  Switch/1 -> Data Store Write3/1
  Data Store Read/1 -> Switch/2

== system Demo/MotionControl/Home/TForAI0 ==
  Action Port : ActionPort  ActionPortLabel=case [ 4 ]:
  Constant1 : Constant  Value=uint16(15)
  Constant3 : Constant  Value=0
  Constant6 : Constant  Value=0
  Constant7 : Constant  Value=uint16(1)
  Data Store Write : DataStoreWrite  DataStoreName=ControlStep  IndexOptions=Index vector (dialog)  Indices=1  OutputSizes=1
  Data Store Write1 : DataStoreWrite  DataStoreName=AI_Enable  IndexOptions=Index vector (dialog)  Indices=1  OutputSizes=1
  Data Store Write2 : DataStoreWrite  DataStoreName=Target_Motor_Acc  IndexOptions=Index vector (dialog)  Indices=1  OutputSizes=1
  Data Store Write3 : DataStoreWrite  DataStoreName=Target_Motor_Current  IndexOptions=Index vector (dialog)  Indices=1  OutputSizes=1
  wires:
  Constant1/1 -> Data Store Write/1
  Constant7/1 -> Data Store Write1/1
  Constant3/1 -> Data Store Write2/1
  Constant6/1 -> Data Store Write3/1

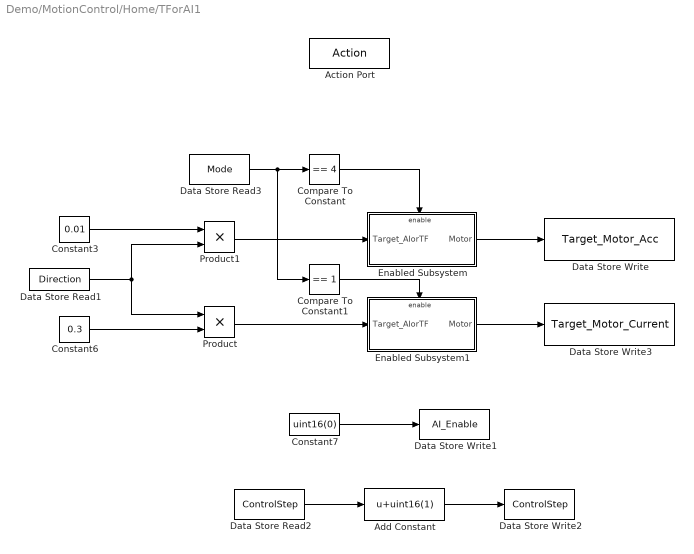
== system Demo/MotionControl/Home/TForAI1 ==
  Action Port : ActionPort  ActionPortLabel=case [ 2 ]:
  Add Constant : Bias  Bias=uint16(1)
  Compare To Constant : simulink/Logic and Bit Operations/Compare To Constant  relop===  const=4  OutDataTypeStr=boolean
  Compare To Constant1 : simulink/Logic and Bit Operations/Compare To Constant  relop===  const=1  OutDataTypeStr=boolean
  Constant3 : Constant  Value=0.01
  Constant6 : Constant  Value=0.3
  Constant7 : Constant  Value=uint16(0)
  Data Store Read1 : DataStoreRead  DataStoreName=Direction  IndexOptions=Index vector (dialog)  Indices=1  OutputSizes=1
  Data Store Read2 : DataStoreRead  DataStoreName=ControlStep  IndexOptions=Index vector (dialog)  Indices=1  OutputSizes=1
  Data Store Read3 : DataStoreRead  DataStoreName=Mode  IndexOptions=Index vector (dialog)  Indices=1  OutputSizes=1
  Data Store Write : DataStoreWrite  DataStoreName=Target_Motor_Acc  IndexOptions=Index vector (dialog)  Indices=1  OutputSizes=1
  Data Store Write1 : DataStoreWrite  DataStoreName=AI_Enable  IndexOptions=Index vector (dialog)  Indices=1  OutputSizes=1
  Data Store Write2 : DataStoreWrite  DataStoreName=ControlStep  IndexOptions=Index vector (dialog)  Indices=1  OutputSizes=1
  Data Store Write3 : DataStoreWrite  DataStoreName=Target_Motor_Current  IndexOptions=Index vector (dialog)  Indices=1  OutputSizes=1
  Enabled Subsystem : Subsystem  TreatAsAtomicUnit=on
  Enabled Subsystem1 : Subsystem  TreatAsAtomicUnit=on
  Product : Product
  Product1 : Product
  wires:
  Data Store Read2/1 -> Add Constant/1
  Add Constant/1 -> Data Store Write2/1
  Data Store Read1/1 -> Product1/2, Product/1
  Constant7/1 -> Data Store Write1/1
  Enabled Subsystem1/1(Motor) -> Data Store Write3/1
  Compare To Constant1/1 -> Enabled Subsystem1/Enable
  Compare To Constant/1 -> Enabled Subsystem/Enable
  Data Store Read3/1 -> Compare To Constant1/1, Compare To Constant/1
  Enabled Subsystem/1(Motor) -> Data Store Write/1
  Product1/1 -> Enabled Subsystem/1(Target_AIorTF)
  Product/1 -> Enabled Subsystem1/1(Target_AIorTF)
  Constant6/1 -> Product/2
  Constant3/1 -> Product1/1

== system Demo/MotionControl/Reset/AI=0 ==
  Action Port : ActionPort  ActionPortLabel=case [ 6 ]:
  AI=100p/s2 : Constant  Value=[hex2dec('4941') 0 1 0]  OutDataTypeStr=uint16
  Add Constant : Bias  Bias=uint16(1)
  Data Store Read : DataStoreRead  DataStoreName=ControlStep  IndexOptions=Index vector (dialog)  Indices=1  OutputSizes=1
  Data Store Write1 : DataStoreWrite  DataStoreName=ControlStep  IndexOptions=Index vector (dialog)  Indices=1  OutputSizes=1
  eCANA Transmit : Subsystem  TreatAsAtomicUnit=on  mask(eCANA Transimit Blocks){MailBoxTx=1, MailBoxRx=4}
      mask help: eCANA MailBox Transimit
      mask DialogControl ParameterGroup Prompt: Parameter Setting
  wires:
  AI=100p/s2/1 -> eCANA Transmit/1(DataTx)
  Add Constant/1 -> Data Store Write1/1
  Data Store Read/1 -> Add Constant/1

== system Demo/MotionControl/Reset/AI=1 ==
  Action Port : ActionPort  ActionPortLabel=case [ 5 ]:
  AI=100p/s2 : Constant  Value=[hex2dec('4941') 1 0 0]  OutDataTypeStr=uint16
  Abs : Abs
  Compare To Constant : simulink/Logic and Bit Operations/Compare To Constant  relop=<=  const=10  OutDataTypeStr=boolean
  Data Type Conversion3 : DataTypeConversion  OutDataTypeStr=int16
  Demux : Demux
  Gain3 : Gain  Gain=0.01  OutDataTypeStr=double
  Subsystem1 : Subsystem
  eCANA Receive : Subsystem  TreatAsAtomicUnit=on  mask(eCANA Transimit Blocks){MailBoxTx=1, MailBoxRx=4}
      mask help: eCANA MailBox Transimit
      mask DialogControl ParameterGroup Prompt: Parameter Setting
  eCANA Transmit : Subsystem  TreatAsAtomicUnit=on  mask(eCANA Transimit Blocks){MailBoxTx=1, MailBoxRx=4}
      mask help: eCANA MailBox Transimit
      mask DialogControl ParameterGroup Prompt: Parameter Setting
  wires:
  AI=100p/s2/1 -> eCANA Transmit/1(DataTx)
  Data Type Conversion3/1 -> Gain3/1
  Demux/3 -> Subsystem1/2(In2)
  Demux/4 -> Subsystem1/3(In3)
  eCANA Receive/1(DataRx) -> Demux/1
  Demux/1 -> Data Type Conversion3/1
  Gain3/1 -> Abs/1, Subsystem1/1(In1)
  Abs/1 -> Compare To Constant/1
  Compare To Constant/1 -> Subsystem1/Enable

== system Demo/MotionControl/Reset/BG  ==
  Action Port : ActionPort  ActionPortLabel=case [ 4 ]:
  Add Constant : Bias  Bias=uint16(1)
  BG : Constant  Value=[hex2dec('4742') 0 0 0]  OutDataTypeStr=uint16
  Data Store Read : DataStoreRead  DataStoreName=ControlStep  IndexOptions=Index vector (dialog)  Indices=1  OutputSizes=1
  Data Store Write1 : DataStoreWrite  DataStoreName=ControlStep  IndexOptions=Index vector (dialog)  Indices=1  OutputSizes=1
  eCANA Transmit : Subsystem  TreatAsAtomicUnit=on  mask(eCANA Transimit Blocks){MailBoxTx=1, MailBoxRx=4}
      mask help: eCANA MailBox Transimit
      mask DialogControl ParameterGroup Prompt: Parameter Setting
  wires:
  BG/1 -> eCANA Transmit/1(DataTx)
  Data Store Read/1 -> Add Constant/1
  Add Constant/1 -> Data Store Write1/1

== system Demo/MotionControl/Reset/JV=0 ==
  Action Port : ActionPort  ActionPortLabel=case [ 7 ]:
  Add Constant : Bias  Bias=uint16(1)
  Data Store Read : DataStoreRead  DataStoreName=ControlStep  IndexOptions=Index vector (dialog)  Indices=1  OutputSizes=1
  Data Store Write1 : DataStoreWrite  DataStoreName=ControlStep  IndexOptions=Index vector (dialog)  Indices=1  OutputSizes=1
  JV : Constant  Value=[hex2dec('564A') 0 0 0]  OutDataTypeStr=uint16
  eCANA Transmit : Subsystem  TreatAsAtomicUnit=on  mask(eCANA Transimit Blocks){MailBoxTx=1, MailBoxRx=4}
      mask help: eCANA MailBox Transimit
      mask DialogControl ParameterGroup Prompt: Parameter Setting
  wires:
  JV/1 -> eCANA Transmit/1(DataTx)
  Data Store Read/1 -> Add Constant/1
  Add Constant/1 -> Data Store Write1/1

== system Demo/MotionControl/Reset/MO=0 ==
  Action Port : ActionPort  ActionPortLabel=case [ 1 ]:
  Add Constant : Bias  Bias=uint16(1)
  Constant2 : Constant  Value=uint16(0)
  Data Store Read : DataStoreRead  DataStoreName=ControlStep  IndexOptions=Index vector (dialog)  Indices=1  OutputSizes=1
  Data Store Write : DataStoreWrite  DataStoreName=Command  IndexOptions=Index vector (dialog)  Indices=1  OutputSizes=1
  Data Store Write1 : DataStoreWrite  DataStoreName=ControlStep  IndexOptions=Index vector (dialog)  Indices=1  OutputSizes=1
  Delay500ms : Subsystem  mask(System Outputs){ShowInLibBrowser=0}
      mask prompts: ShowInLibBrowser "Simulink:masks:CustCodeMaskParam1_MP"
      settings: CopyFcn=cccopyfcn(gcb)  OpenFcn=ccopenfcn('System Outputs Function')
      mask Help: eval('feval(''rtwprivate'',''rtwhelpview'',''rtw_sys_outputs_block'')');
      mask Display: disp('System\nOutputs');
  MO : Constant  Commented=on  Value=[hex2dec('4F4D') 0 0 0]  OutDataTypeStr=uint16
  eCANA Transmit : Subsystem  Commented=on  TreatAsAtomicUnit=on  mask(eCANA Transimit Blocks){MailBoxTx=1, MailBoxRx=4}
      mask help: eCANA MailBox Transimit
      mask DialogControl ParameterGroup Prompt: Parameter Setting
  wires:
  Data Store Read/1 -> Add Constant/1
  MO/1 -> eCANA Transmit/1(DataTx)
  Add Constant/1 -> Data Store Write1/1
  Constant2/1 -> Data Store Write/1

== system Demo/MotionControl/Reset/MO=1 ==
  Action Port : ActionPort  ActionPortLabel=case [ 2 ]:
  Add Constant : Bias  Bias=uint16(1)
  Data Store Read : DataStoreRead  DataStoreName=ControlStep  IndexOptions=Index vector (dialog)  Indices=1  OutputSizes=1
  Data Store Write1 : DataStoreWrite  DataStoreName=ControlStep  IndexOptions=Index vector (dialog)  Indices=1  OutputSizes=1
  Delay500ms : Subsystem  mask(System Outputs){ShowInLibBrowser=0}
      mask prompts: ShowInLibBrowser "Simulink:masks:CustCodeMaskParam1_MP"
      settings: CopyFcn=cccopyfcn(gcb)  OpenFcn=ccopenfcn('System Outputs Function')
      mask Help: eval('feval(''rtwprivate'',''rtwhelpview'',''rtw_sys_outputs_block'')');
      mask Display: disp('System\nOutputs');
  MO : Constant  Value=[hex2dec('4F4D') 0 1 0]  OutDataTypeStr=uint16
  eCANA Transmit : Subsystem  TreatAsAtomicUnit=on  mask(eCANA Transimit Blocks){MailBoxTx=1, MailBoxRx=4}
      mask help: eCANA MailBox Transimit
      mask DialogControl ParameterGroup Prompt: Parameter Setting
  wires:
  Add Constant/1 -> Data Store Write1/1
  MO/1 -> eCANA Transmit/1(DataTx)
  Data Store Read/1 -> Add Constant/1

== system Demo/MotionControl/Reset/PX ==
  Action Port : ActionPort  ActionPortLabel=case [ 8 ]:
  Add Constant : Bias  Bias=uint16(1)
  Data Store Read : DataStoreRead  DataStoreName=ControlStep  IndexOptions=Index vector (dialog)  Indices=1  OutputSizes=1
  Data Store Write1 : DataStoreWrite  DataStoreName=ControlStep  IndexOptions=Index vector (dialog)  Indices=1  OutputSizes=1
  MS : Constant  Commented=on  Value=[hex2dec('5850') 0 0 0]  OutDataTypeStr=uint16
  eCANA Transmit : Subsystem  Commented=on  TreatAsAtomicUnit=on  mask(eCANA Transimit Blocks){MailBoxTx=1, MailBoxRx=4}
      mask help: eCANA MailBox Transimit
      mask DialogControl ParameterGroup Prompt: Parameter Setting
  wires:
  Add Constant/1 -> Data Store Write1/1
  Data Store Read/1 -> Add Constant/1
  MS/1 -> eCANA Transmit/1(DataTx)

== system Demo/MotionControl/Reset/Set_P0 ==
  Action Port : ActionPort  ActionPortLabel=case [ 9 ]:
  Add Constant : Bias  Commented=on  Bias=uint16(1)
  Add1 : Sum  Inputs=+-
  Compare To Constant : simulink/Logic and Bit Operations/Compare To Constant  Commented=on  relop===  const=uint16(hex2dec('5850'))  OutDataTypeStr=boolean
  Constant : Constant  Value=uint16(15)  SampleTime=-1
  Constant1 : Constant  Value=200
  Data Store Read : DataStoreRead  Commented=on  DataStoreName=ControlStep  IndexOptions=Index vector (dialog)  Indices=1  OutputSizes=1
  Data Store Read1 : DataStoreRead  DataStoreName=Motor_Position  IndexOptions=Index vector (dialog)  Indices=1  OutputSizes=1
  Data Store Write1 : DataStoreWrite  Commented=on  DataStoreName=ControlStep  IndexOptions=Index vector (dialog)  Indices=1  OutputSizes=1
  Data Store Write2 : DataStoreWrite  DataStoreName=Motor_Position_Zero  IndexOptions=Index vector (dialog)  Indices=1  OutputSizes=1
  Data Store Write3 : DataStoreWrite  DataStoreName=ControlStep  IndexOptions=Index vector (dialog)  Indices=1  OutputSizes=1
  Demux : Demux  Commented=on
  Enabled Subsystem : Subsystem  Commented=on  TreatAsAtomicUnit=on
  eCANA Receive : Subsystem  Commented=on  TreatAsAtomicUnit=on  mask(eCANA Transimit Blocks){MailBoxTx=1, MailBoxRx=4}
      mask help: eCANA MailBox Transimit
      mask DialogControl ParameterGroup Prompt: Parameter Setting
  wires:
  Demux/1 -> Compare To Constant/1
  Demux/3 -> Enabled Subsystem/1(int_L)
  Compare To Constant/1 -> Enabled Subsystem/Enable
  eCANA Receive/1(DataRx) -> Demux/1
  Demux/4 -> Enabled Subsystem/2(int_H)
  Add Constant/1 -> Data Store Write1/1
  Data Store Read/1 -> Add Constant/1
  Constant1/1 -> Add1/2
  Constant/1 -> Data Store Write3/1
  Add1/1 -> Data Store Write2/1
  Data Store Read1/1 -> Add1/1

== system Demo/MotionControl/Reset/UM=4 ==
  Action Port : ActionPort  ActionPortLabel=case [ 3 ]:
  Add Constant : Bias  Bias=uint16(1)
  Data Store Read : DataStoreRead  DataStoreName=ControlStep  IndexOptions=Index vector (dialog)  Indices=1  OutputSizes=1
  Data Store Write1 : DataStoreWrite  DataStoreName=ControlStep  IndexOptions=Index vector (dialog)  Indices=1  OutputSizes=1
  Delay500ms : Subsystem  mask(System Outputs){ShowInLibBrowser=0}
      mask prompts: ShowInLibBrowser "Simulink:masks:CustCodeMaskParam1_MP"
      settings: CopyFcn=cccopyfcn(gcb)  OpenFcn=ccopenfcn('System Outputs Function')
      mask Help: eval('feval(''rtwprivate'',''rtwhelpview'',''rtw_sys_outputs_block'')');
      mask Display: disp('System\nOutputs');
  UM : Constant  Value=[hex2dec('4D55') 0 4 0]  OutDataTypeStr=uint16
  eCANA Transmit : Subsystem  TreatAsAtomicUnit=on  mask(eCANA Transimit Blocks){MailBoxTx=1, MailBoxRx=4}
      mask help: eCANA MailBox Transimit
      mask DialogControl ParameterGroup Prompt: Parameter Setting
  wires:
  UM/1 -> eCANA Transmit/1(DataTx)
  Data Store Read/1 -> Add Constant/1
  Add Constant/1 -> Data Store Write1/1
